simulink library "INT_RmtAPP_DD2"  (R2016b)
settings: Solver=VariableStepAuto  StartTime=0.0  StopTime=10.0  RelTol=1e-3
settings Model: Creator=xuxingpei  LastModifiedBy=xuxingpei

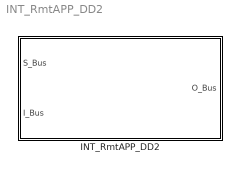
== system INT_RmtAPP_DD2 ==
  INT_RmtAPP_DD2 : Subsystem

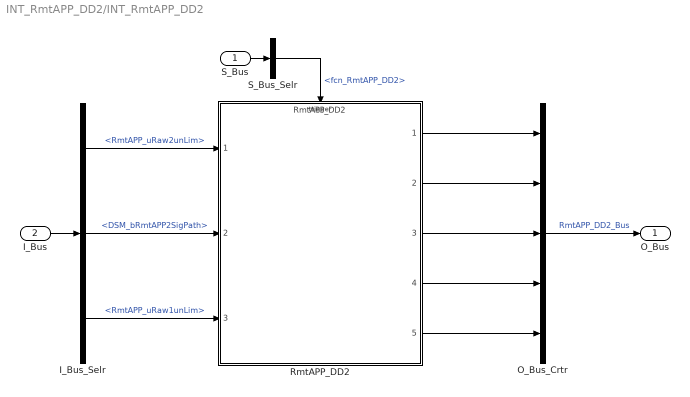
== system INT_RmtAPP_DD2/INT_RmtAPP_DD2 ==
  S_Bus : Inport
  I_Bus : Inport  Port=2
  I_Bus_Selr : BusSelector  OutputSignals=RmtAPP_uRaw2unLim,DSM_bRmtAPP2SigPath,RmtAPP_uRaw1unLim
  O_Bus_Crtr : BusCreator  Inputs=5
  RmtAPP_DD2 : ModelReference  ModelNameDialog=RmtAPP_DD2  SimulationMode=Normal  ModelReferenceVersion=1.19  TriggerPortName=function  TriggerPortTriggerType=function-call  TriggerPortStatesWhenEnabling=held
  S_Bus_Selr : BusSelector  OutputSignals=fcn_RmtAPP_DD2
  O_Bus : Outport
  wires:
  S_Bus_Selr/1 -> RmtAPP_DD2/Trigger  "<fcn_RmtAPP_DD2>"
  S_Bus/1 -> S_Bus_Selr/1
  I_Bus/1 -> I_Bus_Selr/1
  I_Bus_Selr/1 -> RmtAPP_DD2/1  "<RmtAPP_uRaw2unLim>"
  I_Bus_Selr/2 -> RmtAPP_DD2/2  "<DSM_bRmtAPP2SigPath>"
  I_Bus_Selr/3 -> RmtAPP_DD2/3  "<RmtAPP_uRaw1unLim>"
  O_Bus_Crtr/1 -> O_Bus/1  "RmtAPP_DD2_Bus"
  RmtAPP_DD2/1 -> O_Bus_Crtr/1
  RmtAPP_DD2/2 -> O_Bus_Crtr/2
  RmtAPP_DD2/3 -> O_Bus_Crtr/3
  RmtAPP_DD2/4 -> O_Bus_Crtr/4
  RmtAPP_DD2/5 -> O_Bus_Crtr/5
